simulink model "Observador_clasico_plantilla"  (R2016a)
settings: Solver=VariableStepAuto  StartTime=0.0  StopTime=10.0  RelTol=1e-3
values from neighbouring files (symbols this model uses):
  A = [-1,0;0,2]    [Regulador_seguidor_observador_codigo.m]
  B = [1;1]    [Regulador_seguidor_observador_codigo.m]
  C = [1,1]    [Regulador_seguidor_observador_codigo.m]
  ki = k(1:1,3:3)    [Regulador_seguidor_observador_codigo.m]
undefined symbols (not defined in the file or in its folder): denu, deny, numu, numy
settings Model: Creator=Daniel  LastModifiedBy=Daniel

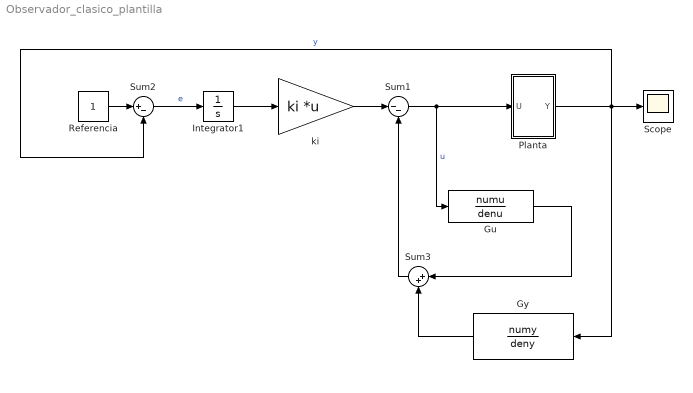
== system Observador_clasico_plantilla ==
  Gu : TransferFcn  Numerator=numu  Denominator=denu
  Gy : TransferFcn  Numerator=numy  Denominator=deny
  Integrator1 : Integrator
  Planta : Subsystem
  Referencia : Constant
  Scope : Scope
  Sum1 : Sum  Inputs=|--
  Sum2 : Sum  Inputs=|+-
  Sum3 : Sum  Inputs=|++
  ki : Gain  Gain=ki  Multiplication=Matrix(K*u) (u vector)
  wires:
  Planta/1(Y) -> Scope/1, Gy/1, Sum2/2  "y"
  Sum1/1 -> Gu/1, Planta/1(U)  "u"
  Integrator1/1 -> ki/1
  Sum2/1 -> Integrator1/1  "e"
  Referencia/1 -> Sum2/1
  ki/1 -> Sum1/1
  Gu/1 -> Sum3/1
  Gy/1 -> Sum3/2
  Sum3/1 -> Sum1/2

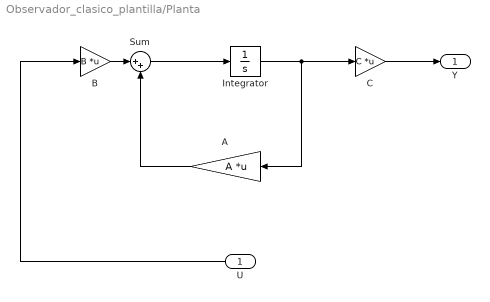
== system Observador_clasico_plantilla/Planta ==
  U : Inport
  A : Gain  Gain=A  Multiplication=Matrix(K*u) (u vector)
  B : Gain  Gain=B  Multiplication=Matrix(K*u) (u vector)
  C : Gain  Gain=C  Multiplication=Matrix(K*u) (u vector)
  Integrator : Integrator
  Sum : Sum  Inputs=|++
  Y : Outport
  wires:
  Sum/1 -> Integrator/1
  A/1 -> Sum/2
  U/1 -> B/1
  B/1 -> Sum/1
  C/1 -> Y/1
  Integrator/1 -> A/1, C/1
